simulink model "Test_actuator"  (R2019b)
settings: Solver=VariableStepAuto  StartTime=0.0  StopTime=tfinal  RelTol=1e-6
undefined symbols (not defined in the file): alpha, Dax, Jm, K_m, Kax, Kcal, Kpad, KR, L_m, L_screw, mu_cal, Mw, N, R_m, X0_caliper
libraries: cstblocks x2
settings Model: Creator=ehsan  LastModifiedBy=ehsan
settings DataIOCC: ReturnWorkspaceOutputs=off
settings DebuggingCC: ArithmeticOperatorsInVariantConditions=warning
settings SFSimCC: SimUseLocalCustomCode=off  CustomCodeUndefinedFunction=UseInterfaceOnly
settings RTWCC: RTWUseLocalCustomCode=off

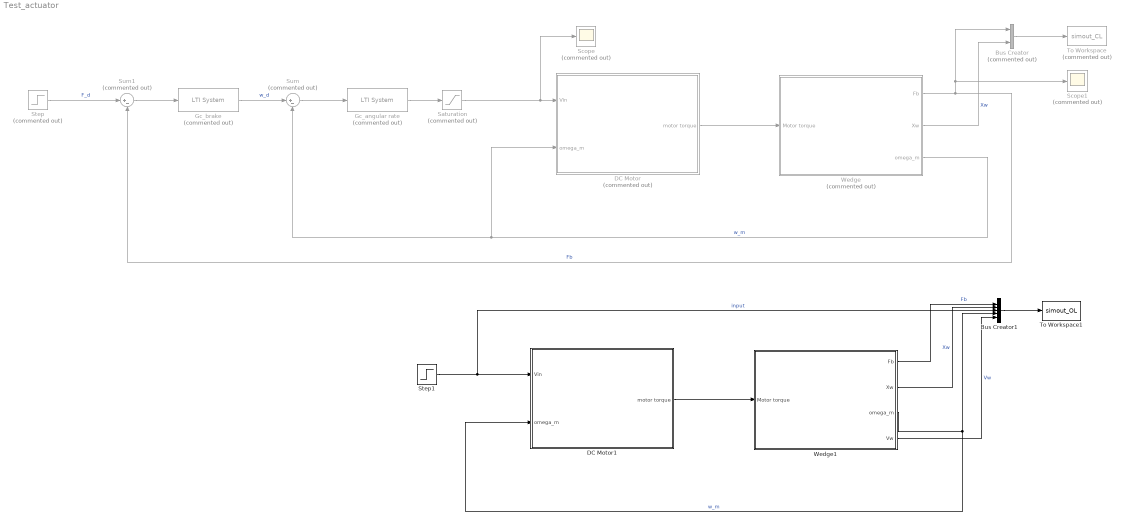
== system Test_actuator ==
  Bus Creator : BusCreator  Commented=on  Inputs=2
  Bus Creator1 : BusCreator  Inputs=5
  DC Motor : Subsystem  Commented=on
  DC Motor1 : Subsystem
  Gc_angular rate : cstblocks/LTI System  Commented=on  sys=Gc_omega  IC=[]
  Gc_brake : cstblocks/LTI System  Commented=on  sys=Gc_brake  IC=[]
  Saturation : Saturate  Commented=on  UpperLimit=100  LowerLimit=-100
  Scope : Scope  Commented=on
  Scope1 : Scope  Commented=on
  Step : Step  Commented=on  Time=0  After=2000  SampleTime=0
  Step1 : Step  Time=0.5  After=12  SampleTime=0
  Sum : Sum  Commented=on  Inputs=|+-
  Sum1 : Sum  Commented=on  Inputs=|+-
  To Workspace : ToWorkspace  Commented=on  VariableName=simout_CL  SaveFormat=Timeseries  SampleTime=-1
  To Workspace1 : ToWorkspace  VariableName=simout_OL  SaveFormat=Timeseries  SampleTime=-1
  Wedge : Subsystem  Commented=on
  Wedge1 : Subsystem
  wires:
  Wedge/2(Xw) -> Bus Creator/2  "Xw"
  DC Motor/1(motor torque) -> Wedge/1(Motor torque)
  Wedge/1(Fb) -> Scope1/1, Bus Creator/1, Sum1/2  "Fb"
  Bus Creator/1 -> To Workspace/1
  Gc_brake/1 -> Sum/1  "w_d"
  Wedge/3(omega_m) -> Sum/2, DC Motor/2(omega_m)  "w_m"
  Sum/1 -> Gc_angular rate/1
  Sum1/1 -> Gc_brake/1
  Step/1 -> Sum1/1  "F_d"
  Wedge1/2(Xw) -> Bus Creator1/2  "Xw"
  Wedge1/1(Fb) -> Bus Creator1/1  "Fb"
  Bus Creator1/1 -> To Workspace1/1
  Wedge1/3(omega_m) -> Bus Creator1/4, DC Motor1/2(omega_m)  "w_m"
  DC Motor1/1(motor torque) -> Wedge1/1(Motor torque)
  Step1/1 -> Bus Creator1/3, DC Motor1/1(Vin)  "input"
  Gc_angular rate/1 -> Saturation/1
  Saturation/1 -> Scope/1, DC Motor/1(Vin)
  Wedge1/4(Vw) -> Bus Creator1/5  "Vw"

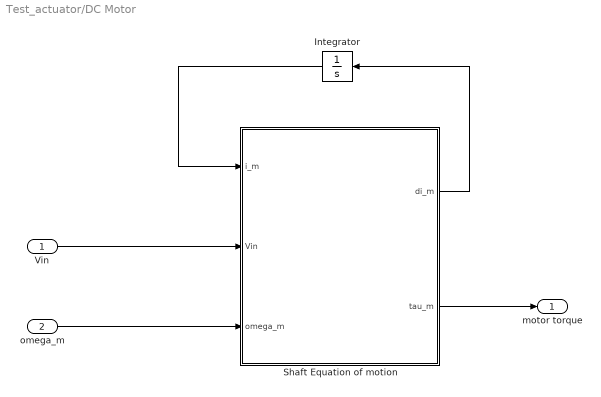
== system Test_actuator/DC Motor ==
  Vin : Inport
  omega_m : Inport  Port=2
  Integrator : Integrator
  Shaft Equation of motion : MATLAB Function  TreatAsAtomicUnit=on
  motor torque : Outport  VectorParamsAs1DForOutWhenUnconnected=off
  wires:
  Integrator/1 -> Shaft Equation of motion/1(i_m)
  Shaft Equation of motion/1(di_m) -> Integrator/1
  Vin/1 -> Shaft Equation of motion/2(Vin)
  omega_m/1 -> Shaft Equation of motion/3(omega_m)
  Shaft Equation of motion/2(tau_m) -> motor torque/1

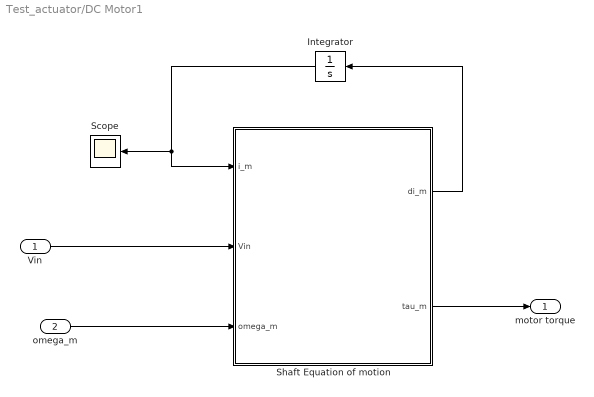
== system Test_actuator/DC Motor1 ==
  Vin : Inport
  omega_m : Inport  Port=2
  Integrator : Integrator
  Scope : Scope
  Shaft Equation of motion : MATLAB Function  TreatAsAtomicUnit=on
  motor torque : Outport  VectorParamsAs1DForOutWhenUnconnected=off
  wires:
  Integrator/1 -> Scope/1, Shaft Equation of motion/1(i_m)
  Shaft Equation of motion/1(di_m) -> Integrator/1
  Vin/1 -> Shaft Equation of motion/2(Vin)
  Shaft Equation of motion/2(tau_m) -> motor torque/1
  omega_m/1 -> Shaft Equation of motion/3(omega_m)

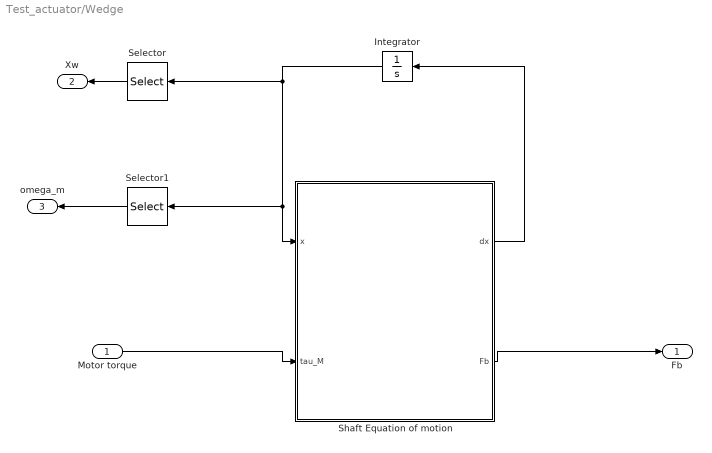
== system Test_actuator/Wedge ==
  Motor torque : Inport
  Integrator : Integrator  InitialCondition=zeros(4,1)  LimitOutput=on  UpperSaturationLimit=[X0_caliper;inf;inf;inf]  LowerSaturationLimit=[0;-inf;-inf;-inf]  WrappedStateUpperValue=[0.5,inf]  WrappedStateLowerValue=[0,-inf]
  Selector : Selector  InputPortWidth=4  IndexOptions=Index vector (dialog)  Indices=[1]  OutputSizes=1
  Selector1 : Selector  InputPortWidth=4  IndexOptions=Index vector (dialog)  Indices=4  OutputSizes=1
  Shaft Equation of motion : MATLAB Function  TreatAsAtomicUnit=on
  Fb : Outport  VectorParamsAs1DForOutWhenUnconnected=off
  Xw : Outport  Port=2  VectorParamsAs1DForOutWhenUnconnected=off
  omega_m : Outport  Port=3  VectorParamsAs1DForOutWhenUnconnected=off
  wires:
  Shaft Equation of motion/2(Fb) -> Fb/1
  Shaft Equation of motion/1(dx) -> Integrator/1
  Integrator/1 -> Selector/1, Selector1/1, Shaft Equation of motion/1(x)
  Motor torque/1 -> Shaft Equation of motion/2(tau_M)
  Selector/1 -> Xw/1
  Selector1/1 -> omega_m/1

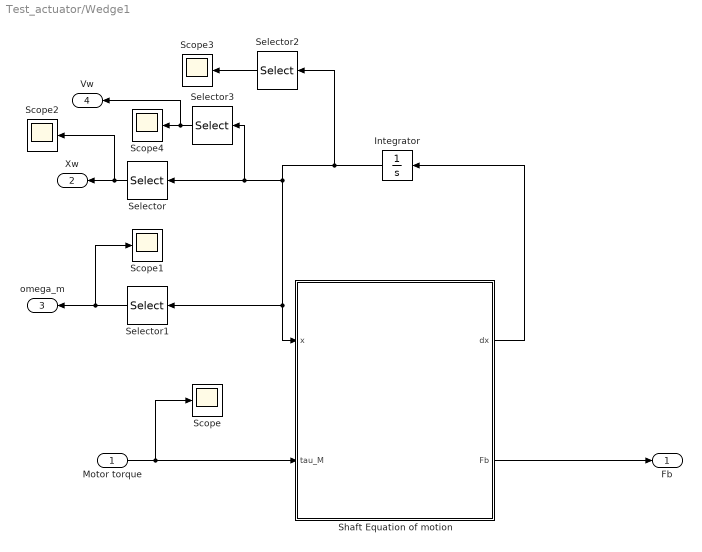
== system Test_actuator/Wedge1 ==
  Motor torque : Inport
  Integrator : Integrator  InitialCondition=zeros(5,1)  LimitOutput=on  UpperSaturationLimit=[inf;inf;inf;X0_caliper;inf]  LowerSaturationLimit=[-inf;-inf;-inf;0;-inf]  WrappedStateUpperValue=[0.5,inf]  WrappedStateLowerValue=[0,-inf]
  Scope{,1..4} (5 alike) : Scope
  Selector : Selector  InputPortWidth=5  IndexOptions=Index vector (dialog)  Indices=4  OutputSizes=1
  Selector1 : Selector  InputPortWidth=5  IndexOptions=Index vector (dialog)  Indices=1  OutputSizes=1
  Selector2 : Selector  InputPortWidth=5  IndexOptions=Index vector (dialog)  Indices=2  OutputSizes=1
  Selector3 : Selector  InputPortWidth=5  IndexOptions=Index vector (dialog)  Indices=3  OutputSizes=1
  Shaft Equation of motion : MATLAB Function  TreatAsAtomicUnit=on
  Fb : Outport  VectorParamsAs1DForOutWhenUnconnected=off
  Xw : Outport  Port=2  VectorParamsAs1DForOutWhenUnconnected=off
  omega_m : Outport  Port=3  VectorParamsAs1DForOutWhenUnconnected=off
  Vw : Outport  Port=4  VectorParamsAs1DForOutWhenUnconnected=off
  wires:
  Shaft Equation of motion/2(Fb) -> Fb/1
  Shaft Equation of motion/1(dx) -> Integrator/1
  Integrator/1 -> Selector2/1, Selector3/1, Selector/1, Selector1/1, Shaft Equation of motion/1(x)
  Motor torque/1 -> Scope/1, Shaft Equation of motion/2(tau_M)
  Selector1/1 -> Scope1/1, omega_m/1
  Selector/1 -> Scope2/1, Xw/1
  Selector2/1 -> Scope3/1
  Selector3/1 -> Vw/1, Scope4/1

== matlab function Test_actuator/Wedge/Shaft Equation of motion ==
  data: dx output; x input; Fb output; tau_M input; alpha parameter; Mw parameter; Kcal parameter; mu_cal parameter; Jm parameter; L_screw parameter; Kax parameter; Dax parameter
function [dx,Fb] = fcn(x,tau_M,alpha, Mw, Kcal, mu_cal, Jm, ...
    L_screw, Kax, Dax)


Xw = x(1);
Vw = x(2); 
theta = x(3);
omega = x(4);


dtheta = omega;
domega = 1/Jm * (tau_M);


L = L_screw;

%F_M = -L/(2*pi) * 1/eta * (Kax*(Xw-theta*L/(2*pi*cos(alpha)))+...
 %    Dax*(Vw-omega*L/(2*pi*cos(alpha))));

F_M =  -(Kax*(Xw/cos(alpha)-theta*L/(2*pi))-...
         Dax*(Vw/cos(alpha)-omega*L/(2*pi)));



A1 = 1/(Mw*(1+tan(alpha)^2))*1/cos(alpha);
B1 = ((mu_cal-tan(alpha))*Kcal*tan(alpha))/(Mw*(1+tan(alpha)^2));

dVw = A1*F_M + B1* Xw;
dXw = Vw;


Fb = mu_cal*Kcal*Xw*tan(alpha);

dx = [dXw;dVw;dtheta;domega];

== matlab function Test_actuator/DC Motor/Shaft Equation of motion ==
  data: di_m output; i_m input; Vin input; omega_m input; L_m parameter; K_m parameter; R_m parameter; tau_m output
function [di_m,tau_m]  = fcn(i_m,Vin,omega_m,L_m,K_m, R_m)



di_m = 1/L_m * (Vin-i_m*R_m-K_m*omega_m);


tau_m = K_m * i_m;

%T_M = -L/(2*pi) * (K_ax*(X_w-theta*L/(2*pi*cos(alpha)))+...
%    D_ax * (V_w-omega_m*L/(2*pi*cos(alpha)))) * 1/eta;

== matlab function Test_actuator/DC Motor1/Shaft Equation of motion ==
  data: di_m output; i_m input; Vin input; omega_m input; L_m parameter; K_m parameter; R_m parameter; tau_m output
function [di_m,tau_m]  = fcn(i_m,Vin,omega_m,L_m,K_m, R_m)



di_m = 1/L_m * (Vin-i_m*R_m-K_m*omega_m);


tau_m = K_m * i_m;

== matlab function Test_actuator/Wedge1/Shaft Equation of motion ==
  data: dx output; x input; Fb output; tau_M input; alpha parameter; Mw parameter; Kcal parameter; mu_cal parameter; Jm parameter; L_screw parameter; Kax parameter; Dax parameter; N parameter; KR parameter; Kpad parameter
function [dx,Fb] = fcn(x,tau_M,alpha, Mw, Kcal, mu_cal, Jm, ...
    L_screw,Kax, Dax,N,KR, Kpad)


omega = x(1);
qax = x(2); 
Vw = x(3);
qpad = x(4);
qR = x(5);


T1 = sin(alpha)/tan(alpha)+cos(alpha);
T2 = -cos(alpha)/tan(alpha)+sin(alpha);
T3 = (tan(alpha)*mu_cal + 1);

domega = 1/Jm * (tau_M - L_screw*N/(2*pi)*(Kax*qax+Dax*(L_screw*N/(2*pi))*omega-...
    (2/T1)*Vw));
dqax = L_screw*N/(2*pi) * omega - (2/T1) * Vw;
dVw = 1/(2*Mw) * (-T2*KR*qR...
                  +T1*(Kax*qax+Dax*(L_screw*N/(2*pi)*omega-(2/T1)*Vw))...
                  -T3*(Kcal+Kpad)*qpad...
                  -Kpad*qpad);
dqpad = T3 * Vw;
dqR = T2 * Vw;


Fb = mu_cal*Kpad*qpad*tan(alpha);

dx = [domega;dqax;dVw;dqpad;dqR];

% Xw = x(1);
% Vw = x(2); 
% theta = x(3);
% omega = x(4);
% 
% a3 = cos(alpha);
% a4 = L_screw*N/(2*pi);
% T1 = a4*Kax/(eta*a3) * Xw +  a4*Dax/(eta*a3) * Vw - (a4^2*Kax/eta...
%     + a4^2*Dax/eta)*theta ;
% 
% 
% dtheta = omega;
% domega = 1/Jm * (tau_M) - Dm/Jm * omega + 1/Jm * T1;
% 
% 
% L = L_screw;
% 
% %F_M = -L/(2*pi) * 1/eta * (Kax*(Xw-theta*L/(2*pi*cos(alpha)))+...
%  %    Dax*(Vw-omega*L/(2*pi*cos(alpha))));
% 
% F_M =  -(Kax*(Xw/cos(alpha)-theta*L*N/(2*pi))-...
%          Dax*(Vw/cos(alpha)-omega*L*N/(2*pi)));
% 
% 
% 
% A1 = 1/(Mw*(1+tan(alpha)^2))*1/cos(alpha);
% B1 = ((mu_cal-tan(alpha))*Kcal*tan(alpha))/(Mw*(1+tan(alpha)^2));
% 
% dVw = A1*F_M + B1* Xw;
% dXw = Vw;
% 
% 
% Fb = mu_cal*Kcal*Xw*tan(alpha);
% 
% dx = [dXw;dVw;dtheta;domega];
